simulink model "sintester"  (R2016a)
settings: Solver=VariableStepAuto  StartTime=0.0  StopTime=100.0  RelTol=1e-6
libraries: simulink x1
settings Model: Creator=tommi  LastModifiedBy=tommi

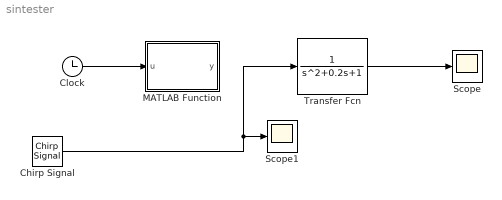
== system sintester ==
  Chirp Signal : simulink/Sources/Chirp Signal  f1=0.0  T=100  f2=1
  Clock : Clock
  MATLAB Function : MATLAB Function  TreatAsAtomicUnit=on
  Scope : Scope
  Scope1 : Scope
  Transfer Fcn : TransferFcn  Denominator=[1 0.2 1]
  wires:
  Clock/1 -> MATLAB Function/1(u)
  Transfer Fcn/1 -> Scope/1
  Chirp Signal/1 -> Scope1/1, Transfer Fcn/1

== matlab function sintester/MATLAB Function ==
  data: u input; y output
function y = fcn(u)
y = sin(u);
end
